simulink library "movingAverage_1ms_to_5ms"  (R2016b)
settings: Solver=VariableStepAuto  StartTime=0.0  StopTime=10.0  RelTol=1e-3
settings Model: Creator=oelkawok  LastModifiedBy=oelkawok

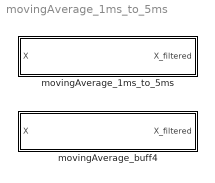
== system movingAverage_1ms_to_5ms ==
  movingAverage_1ms_to_5ms : Subsystem
  movingAverage_buff4 : Subsystem

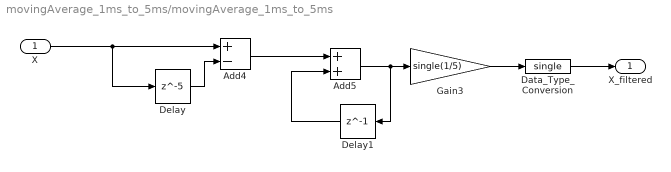
== system movingAverage_1ms_to_5ms/movingAverage_1ms_to_5ms ==
  X : Inport
  Add4 : Sum  Inputs=+-
  Add5 : Sum
  Data_Type_Conversion : DataTypeConversion  OutDataTypeStr=single
  Delay : Delay  DelayLength=5
      settings: AttributesFormatString=Init: %<InitialCondition>
  Delay1 : Delay  DelayLength=1  InitialCondition=single(0)
      settings: AttributesFormatString=Init: %<InitialCondition>
  Gain3 : Gain  Gain=single(1/5)
  X_filtered : Outport
  wires:
  Add4/1 -> Add5/1
  Add5/1 -> Delay1/1, Gain3/1
  Delay1/1 -> Add5/2
  Delay/1 -> Add4/2
  Gain3/1 -> Data_Type_Conversion/1
  X/1 -> Add4/1, Delay/1
  Data_Type_Conversion/1 -> X_filtered/1

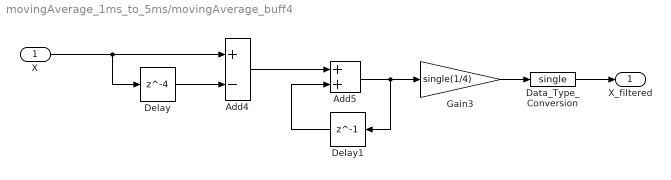
== system movingAverage_1ms_to_5ms/movingAverage_buff4 ==
  X : Inport
  Add4 : Sum  Inputs=+-
  Add5 : Sum
  Data_Type_Conversion : DataTypeConversion  OutDataTypeStr=single
  Delay : Delay  DelayLength=4
      settings: AttributesFormatString=Init: %<InitialCondition>
  Delay1 : Delay  DelayLength=1  InitialCondition=single(0)
      settings: AttributesFormatString=Init: %<InitialCondition>
  Gain3 : Gain  Gain=single(1/4)
  X_filtered : Outport
  wires:
  Data_Type_Conversion/1 -> X_filtered/1
  X/1 -> Delay/1, Add4/1
  Gain3/1 -> Data_Type_Conversion/1
  Delay/1 -> Add4/2
  Delay1/1 -> Add5/2
  Add5/1 -> Gain3/1, Delay1/1
  Add4/1 -> Add5/1
